simulink model "simulinkPBLextended"  (R2020b)
settings: Solver=VariableStepAuto  StartTime=0.0  StopTime=100000  RelTol=1e-3
model workspace (MAT data in the model file):
  ON_OFF = 0
  SL_ROS_VariableLengthArrays_MaxSizes : object (value not decoded)
values from neighbouring files (symbols this model uses):
  distToReach = 0.1    [scriptPBLextended.m]
  mapSize = zeros(7,7)    [scriptPBLextended.m]
  myGoals = [  2.5   1  1;                0.2   1   0]    [scriptPBLextended.m]
  slow_ang = 0.2    [scriptPBLextended.m]
  slow_vel = 0.2    [scriptPBLextended.m]
  vizLim = [5;5;0;0]    [scriptPBLextended.m]
undefined symbols (not defined in the file or in its folder): Angular, Linear
libraries: robotlib x9, robotalgslib x2, robotcorelib x1
(part 2 of 3)

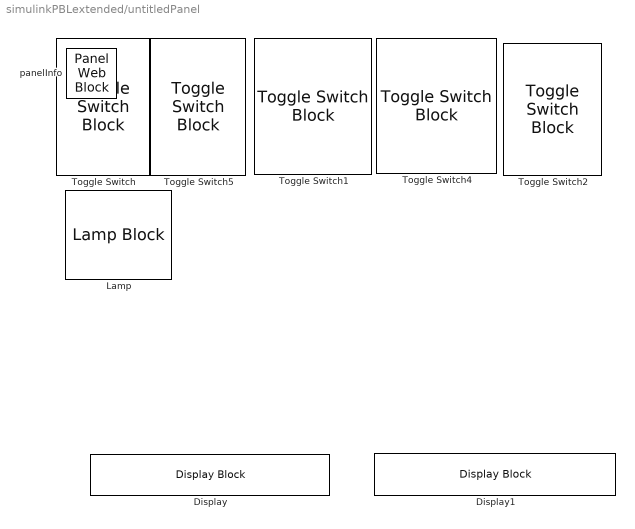
== system simulinkPBLextended/untitledPanel ==
  Display : DisplayBlock  Tag=HiddenForWebPanel  PanelInfo="{\"panelId\":\"panelId-ee0204e8-1368-44d2-ae33-7b337b0ca082\",\"type\":\"panelChild\",\"version\":\"2019b\",\"zIndex\":1500008}"  Format=short  Transparency=1
  Display1 : DisplayBlock  Tag=HiddenForWebPanel  PanelInfo="{\"panelId\":\"panelId-ee0204e8-1368-44d2-ae33-7b337b0ca082\",\"type\":\"panelChild\",\"version\":\"2019b\",\"zIndex\":1500010}"  Format=short  Transparency=1
  Lamp : LampBlock  Tag=HiddenForWebPanel  PanelInfo="{\"panelId\":\"panelId-ee0204e8-1368-44d2-ae33-7b337b0ca082\",\"type\":\"panelChild\",\"version\":\"2019b\",\"zIndex\":1500030}"
  Toggle Switch : ToggleSwitchBlock  Tag=HiddenForWebPanel  PanelInfo="{\"panelId\":\"panelId-ee0204e8-1368-44d2-ae33-7b337b0ca082\",\"type\":\"panelChild\",\"version\":\"2019b\",\"zIndex\":1500014}"  LabelPosition=Hide
      settings: Values={{'Steering Off', 'Steering On'}, [0 1]}
  Toggle Switch1 : ToggleSwitchBlock  Tag=HiddenForWebPanel  PanelInfo="{\"panelId\":\"panelId-ee0204e8-1368-44d2-ae33-7b337b0ca082\",\"type\":\"panelChild\",\"version\":\"2019b\",\"zIndex\":1500016}"  LabelPosition=Hide
      settings: Values={{'Do nothing', 'Send "True" to Arm'}, [0 1]}
  Toggle Switch2 : ToggleSwitchBlock  Tag=HiddenForWebPanel  PanelInfo="{\"panelId\":\"panelId-ee0204e8-1368-44d2-ae33-7b337b0ca082\",\"type\":\"panelChild\",\"version\":\"2019b\",\"zIndex\":1500012}"  LabelPosition=Hide
      settings: Values={{'Real Platform', 'Simulation'}, [0 1]}
  Toggle Switch4 : ToggleSwitchBlock  Tag=HiddenForWebPanel  PanelInfo="{\"panelId\":\"panelId-ee0204e8-1368-44d2-ae33-7b337b0ca082\",\"type\":\"panelChild\",\"version\":\"2019b\",\"zIndex\":1500028}"  LabelPosition=Hide
      settings: Values={{'Info zPlatformy', 'Wyślij Załadowany'}, [0 1]}
  Toggle Switch5 : ToggleSwitchBlock  Tag=HiddenForWebPanel  PanelInfo="{\"panelId\":\"panelId-ee0204e8-1368-44d2-ae33-7b337b0ca082\",\"type\":\"panelChild\",\"version\":\"2019b\",\"zIndex\":1500026}"  LabelPosition=Hide
      settings: Values={{'Off', 'Backward ON'}, [0 1]}
  panelInfo : PanelWebBlock  Tag=HiddenForWebPanel  PanelInfo="{\"compacted\":true,\"height\":493,\"left\":-2,\"name\":\"untitledPanel\",\"panelId\":\"panelId-ee0204e8-1368-44d2-ae33-7b337b0ca082\",\"top\":-6,\"type\":\"panel\",\"version\":\"2019b\",\"visible\":true,\"width\":601,\"zIndex\":1500002}"  PanelSnapshot=<binary blob, 330192 chars, not shown>  PanelBackground=data:image/jpeg;base64,/9j/4AAQSkZJRgABAQAAAQABAAD/2wBDAAMCAggICAgICAgICAgICAgICAgICAgICAgICAgICAgICAgICAgICAgICAgICAoICAgICQkJCAgNDQoIDQgICQj/2wBDAQMEBAYFBggGBggICAgHCAgICAgICAgICAgICAgICAgICAgICAgICAgICAgICAgICAgICAgICAgICAgICAgICAj/wgARCAQrBkADASIAAhEBAxEB/8QAHAAAAwADAQEBAAAAAAAAAAAAAAECAwQFBgcI/8QAGAEBAQEBAQAAAAAAAAAAAAAAAAECAwT/2gAMAwEAAhADEAAAAfnaaATBBANADAagEwTBDAABgAMTGIYAMQwRQS2CbBDBDZLYIYIYIbEqQDBDBDCWwkoEMEME ...(+234152 chars)
